simulink model "Project5"  (R2016a)
settings: Solver=ode5  StartTime=0.0  StopTime=10.0  FixedStep=0.01  RelTol=1e-3
values from neighbouring files (symbols this model uses):
  Kd = 0.1    [Project5_Code.m]
  Ki = 1    [Project5_Code.m]
  Kp = 1    [Project5_Code.m]
  sw = 0    [Project5_Code.m]
settings Model: Creator=Dell  LastModifiedBy=Dell

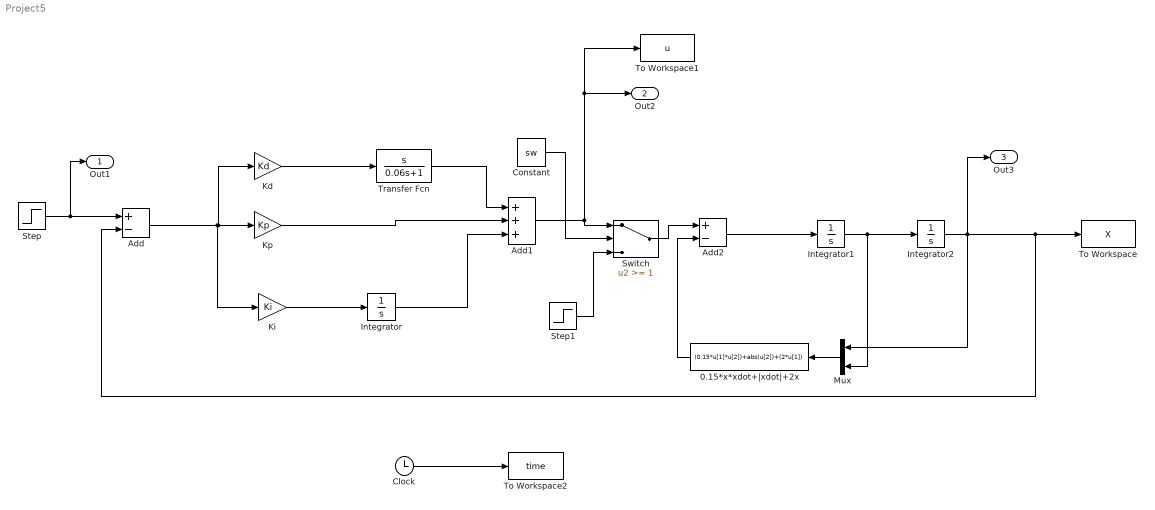
== system Project5 ==
  0.15*x*xdot+|xdot|+2x : Fcn  Expr=(0.15*u[1]*u[2])+abs(u[2])+(2*u[1])
  Add : Sum  Inputs=+-
  Add1 : Sum  Inputs=+++
  Add2 : Sum  Inputs=+-
  Clock : Clock
  Constant : Constant  Value=sw
  Integrator : Integrator
  Integrator1 : Integrator
  Integrator2 : Integrator
  Kd : Gain  Gain=Kd
  "Ki " : Gain  Gain=Ki
  Kp : Gain  Gain=Kp
  Mux : Mux  Inputs=2
  Step : Step  Time=0  SampleTime=0
  Step1 : Step  Time=0  SampleTime=0
  Switch : Switch  Threshold=1
  To Workspace : ToWorkspace  VariableName=X  SampleTime=-1
  To Workspace1 : ToWorkspace  VariableName=u  SampleTime=-1
  To Workspace2 : ToWorkspace  VariableName=time  SampleTime=-1
  Transfer Fcn : TransferFcn  Numerator=[1 0]  Denominator=[0.06 1]
  Out1 : Outport
  Out2 : Outport  Port=2
  Out3 : Outport  Port=3
  wires:
  Step/1 -> Add/1, Out1/1
  Add/1 -> "Ki "/1, Kd/1, Kp/1
  "Ki "/1 -> Integrator/1
  Kd/1 -> Transfer Fcn/1
  Kp/1 -> Add1/2
  Transfer Fcn/1 -> Add1/1
  Integrator/1 -> Add1/3
  Add1/1 -> Out2/1, To Workspace1/1, Switch/1
  Add2/1 -> Integrator1/1
  Integrator1/1 -> Mux/2, Integrator2/1
  Integrator2/1 -> Out3/1, Mux/1, Add/2, To Workspace/1
  Mux/1 -> 0.15*x*xdot+|xdot|+2x/1
  0.15*x*xdot+|xdot|+2x/1 -> Add2/2
  Clock/1 -> To Workspace2/1
  Switch/1 -> Add2/1
  Constant/1 -> Switch/2
  Step1/1 -> Switch/3
